simulink model "PthLead_TrqCalc"  (R2016b)
settings: configuration reference "CodeGenConfigSet" (kept outside this file)
values from neighbouring files (symbols this model uses):
  TRQ_ZERO = fi(0,Trq_Nm)    [init_PthLead_TrqCalc.m]    (also in init_PthLead_TrqCalc_SIL.m)
undefined symbols (not defined in the file or in its folder): EngState_conv
libraries: simulink x6
settings Model: Creator=Wollf  LastModifiedBy=xuxingpei
settings ConfigSetRef: SourceLocation=Base Workspace

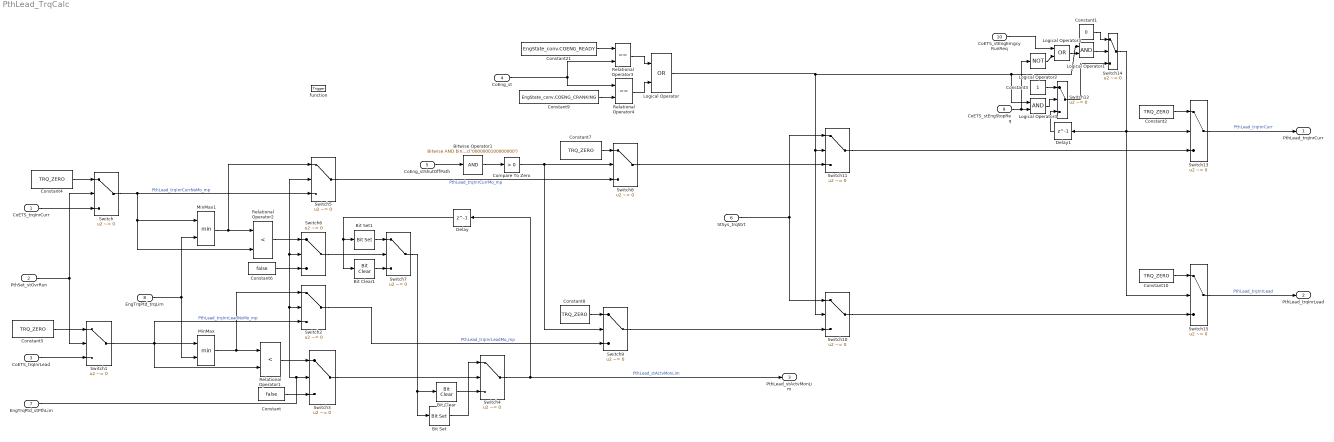
== system PthLead_TrqCalc ==
  CoETS_trqInrCurr : Inport  Tag=Nm  Description=Inner torque current value  OutMin=-3276  OutMax=3276  OutDataTypeStr=Trq_Nm
  PthSet_stOvrRun : Inport  Description=State of overrun detection (0: No overrun; 1: overrun)  Port=2  OutMin=0  OutMax=1  OutDataTypeStr=boolean
  CoETS_trqInrLead : Inport  Tag=Nm  Description=desired lead (inner) torque (without Filter with reserve)  Port=3  OutMin=-3276  OutMax=3276  OutDataTypeStr=Trq_Nm
  CoEng_st : Inport  Description=Engine coordinator state  Port=4  OutDataTypeStr=Enum: EngState_conv
  CoEng_stShutOffPath : Inport  Description=Active shut-off paths resulting from active reversible,irreversible and afterrun shut-off paths  Port=5  OutMin=0  OutMax=65535  OutDataTypeStr=State_uint16
  StSys_trqStrt : Inport  Tag=Nm  Description=Engine starting torque  Port=6  OutMin=-3000  OutMax=3000  OutDataTypeStr=Trq_Nm
  EngTrqPtd_stPthLim : Inport  Description=State of engine torque limitation from ECU monitoring  Port=7  OutMin=0  OutMax=255  OutDataTypeStr=State_uint8
  EngTrqPtd_trqLim : Inport  Tag=Nm  Description=Set path torque limitation from ECU monitoring  Port=8  OutMin=-3276  OutMax=3276  OutDataTypeStr=Trq_Nm
  CoETS_stEngStopReq : Inport  Description=Tbox Engine stop request  Port=9  OutMin=0  OutMax=1  OutDataTypeStr=boolean
  CoETS_stEngEmgcyRunReq : Inport  Description=Tbox Engine emergency start request  Port=10  OutMin=0  OutMax=1  OutDataTypeStr=boolean
  function : TriggerPort  TriggerType=function-call  VariantControl=Variant
  Bit Clear : simulink/Logic and Bit Operations/Bit Clear  iBit=1
  Bit Clear1 : simulink/Logic and Bit Operations/Bit Clear  iBit=0
  Bit Set : simulink/Logic and Bit Operations/Bit Set  iBit=1
  Bit Set1 : simulink/Logic and Bit Operations/Bit Set  iBit=0
  Bitwise Operator1 : simulink/Logic and Bit Operations/Bitwise Operator  logicop=AND  UseBitMask=on  BitMask=bin2dec('0000000100000000')  BitMaskRealWorld=Stored Integer
  Compare To Zero : simulink/Logic and Bit Operations/Compare To Zero  relop=>  OutDataTypeStr=boolean
  Constant : Constant  Value=false  OutDataTypeStr=boolean
  Constant1 : Constant  Value=0  OutDataTypeStr=Inherit: Inherit via back propagation
  Constant{2,4..5,7..8,10} (6 alike) : Constant  Value=TRQ_ZERO  OutDataTypeStr=Inherit: Inherit via back propagation
  Constant21 : Constant  Value=EngState_conv.COENG_READY  OutDataTypeStr=Inherit: Inherit via back propagation
  Constant3 : Constant  OutDataTypeStr=Inherit: Inherit via back propagation
  Constant6 : Constant  Value=false  OutDataTypeStr=boolean
  Constant9 : Constant  Value=EngState_conv.COENG_CRANKING  OutDataTypeStr=Inherit: Inherit via back propagation
  Delay : Delay  DelayLength=1  InitialCondition=0
  Delay1 : Delay  DelayLength=1  InitialCondition=0
  Logical Operator : Logic  Operator=OR  OutDataTypeStr=boolean
  Logical Operator1 : Logic  AllPortsSameDT=off  OutDataTypeStr=boolean
  Logical Operator2 : Logic  Operator=NOT  AllPortsSameDT=off  OutDataTypeStr=boolean
  Logical Operator3 : Logic  Operator=OR  AllPortsSameDT=off  OutDataTypeStr=boolean
  Logical Operator4 : Logic  AllPortsSameDT=off  OutDataTypeStr=boolean
  MinMax : MinMax  Inputs=2  InputSameDT=on
  MinMax1 : MinMax  Inputs=2  InputSameDT=on
  Relational Operator1 : RelationalOperator  Operator=<  OutDataTypeStr=boolean  RndMeth=Simplest  InputSameDT=on
  Relational Operator2 : RelationalOperator  Operator=<  OutDataTypeStr=boolean  RndMeth=Simplest  InputSameDT=on
  Relational Operator3 : RelationalOperator  Operator===  OutDataTypeStr=boolean  RndMeth=Simplest  InputSameDT=on
  Relational Operator4 : RelationalOperator  Operator===  OutDataTypeStr=boolean  RndMeth=Simplest  InputSameDT=on
  Switch{,1..11,13,15} (14 alike) : Switch  Criteria=u2 ~= 0  InputSameDT=on
  Switch12 : Switch  Criteria=u2 ~= 0
  Switch14 : Switch  Criteria=u2 ~= 0
  PthLead_trqInrCurr : Outport  Tag=Nm  Description=Actual percent engine torque  OutMin=-3000  OutMax=3000  OutDataTypeStr=Trq_Nm
  PthLead_trqInrLead : Outport  Tag=Nm  Description=Inner torque lead value  Port=2  OutMin=-3000  OutMax=3000  OutDataTypeStr=Trq_Nm
  PthLead_stActvMonLim : Outport  Description=State of monitoring limitation  Port=3  OutMin=0  OutMax=255  OutDataTypeStr=State_uint8
  wires:
  Constant4/1 -> Switch/1
  CoETS_trqInrCurr/1 -> Switch/3
  Switch/1 -> Switch5/3, MinMax1/1, Relational Operator2/2  "PthLead_trqInrCurrNoMo_mp"
  CoETS_trqInrLead/1 -> Switch1/3
  Constant5/1 -> Switch1/1
  PthSet_stOvrRun/1 -> Switch1/2, Switch/2
  Switch1/1 -> Relational Operator1/2, MinMax/1, Switch2/3  "PthLead_trqInrLeadNoMo_mp"
  MinMax/1 -> Relational Operator1/1, Switch2/1
  EngTrqPtd_trqLim/1 -> MinMax/2, MinMax1/2
  Relational Operator1/1 -> Switch3/1
  Constant/1 -> Switch3/3
  Switch3/1 -> Switch4/2
  Switch4/1 -> PthLead_stActvMonLim/1, Delay/1  "PthLead_stActvMonLim"
  Bit Set/1 -> Switch4/1
  Bit Clear/1 -> Switch4/3
  EngTrqPtd_stPthLim/1 -> Switch5/2, Switch6/2, Switch2/2, Switch3/2
  MinMax1/1 -> Switch5/1, Relational Operator2/1
  Relational Operator2/1 -> Switch6/1
  Constant6/1 -> Switch6/3
  Switch6/1 -> Switch7/2
  Bit Set1/1 -> Switch7/1
  Bit Clear1/1 -> Switch7/3
  Switch7/1 -> Bit Set/1, Bit Clear/1
  Delay/1 -> Bit Set1/1, Bit Clear1/1
  CoEng_stShutOffPath/1 -> Bitwise Operator1/1
  Bitwise Operator1/1 -> Compare To Zero/1
  Switch5/1 -> Switch8/3  "PthLead_trqInrCurrMo_mp"
  Switch2/1 -> Switch9/3  "PthLead_trqInrLeadMo_mp"
  Constant7/1 -> Switch8/1
  Constant8/1 -> Switch9/1
  Switch9/1 -> Switch10/3
  Switch8/1 -> Switch11/3
  StSys_trqStrt/1 -> Switch11/1, Switch10/1
  CoEng_st/1 -> Relational Operator3/2, Relational Operator4/1
  Constant21/1 -> Relational Operator3/1
  Constant9/1 -> Relational Operator4/2
  Relational Operator3/1 -> Logical Operator/1
  Relational Operator4/1 -> Logical Operator/2
  Compare To Zero/1 -> Switch8/2, Switch9/2
  Logical Operator/1 -> Switch11/2, Switch10/2, Logical Operator4/1, Logical Operator1/1
  Switch11/1 -> Switch13/3
  Switch13/1 -> PthLead_trqInrCurr/1  "PthLead_trqInrCurr"
  Constant2/1 -> Switch13/1
  Switch12/1 -> Switch14/3
  Constant1/1 -> Switch14/1
  Constant3/1 -> Switch12/1
  Logical Operator1/1 -> Switch14/2
  Logical Operator2/1 -> Logical Operator3/2
  Logical Operator3/1 -> Logical Operator1/2
  CoETS_stEngEmgcyRunReq/1 -> Logical Operator3/1
  Logical Operator4/1 -> Switch12/2
  CoETS_stEngStopReq/1 -> Logical Operator2/1, Logical Operator4/2
  Delay1/1 -> Switch12/3
  Switch10/1 -> Switch15/3
  Switch15/1 -> PthLead_trqInrLead/1  "PthLead_trqInrLead"
  Constant10/1 -> Switch15/1
  Switch14/1 -> Switch15/2, Delay1/1, Switch13/2
